simulink model "ex_4"  (R2023b)
settings: Solver=VariableStepAuto  StartTime=0.0  StopTime=10.0  RelTol=1e-3
settings Model: Creator=LucasDaiPráMartens  LastModifiedBy=LucasDaiPráMartens

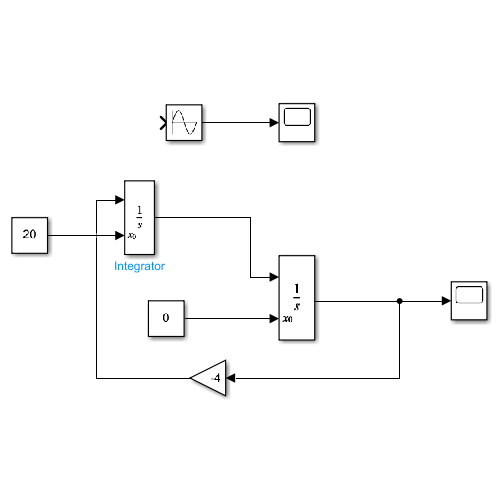
[thumbnail: Simulink's stored preview of the top-level diagram]
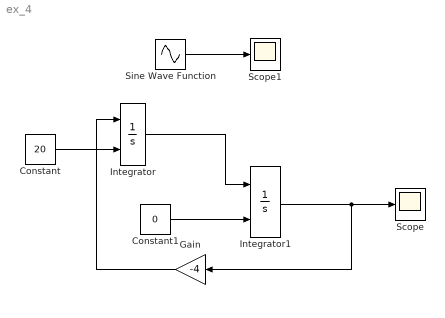
== system ex_4 ==
  Constant : Constant  Value=20
  Constant1 : Constant  Value=0
  Gain : Gain  Gain=-4
  Integrator : Integrator  InitialConditionSource=external
  Integrator1 : Integrator  InitialConditionSource=external
  Scope : Scope
  Scope1 : Scope
  Sine Wave Function : Sin  TimeSource=Use external signal  Amplitude=10  Frequency=2  SampleTime=0
  wires:
  Constant/1 -> Integrator/2
  Constant1/1 -> Integrator1/2
  Integrator1/1 -> Scope/1, Gain/1
  Integrator/1 -> Integrator1/1
  Gain/1 -> Integrator/1
  Sine Wave Function/1 -> Scope1/1
